simulink model "PriOrdemZero"  (R2015a)
settings: Solver=ode45  StartTime=0.0  StopTime=50  FixedStep=1e-8  RelTol=1e-5
settings Model: Creator=user  LastModifiedBy=user
settings SolverCC: ZeroCrossAlgorithm=Adaptive
settings OptimizationCC: BlockReduction=off  OptimizeBlockIOStorage=off  BufferReuse=off  GlobalBufferReuse=off  ExpressionFolding=off  LocalBlockOutputs=off
settings DebuggingCC: ConsistencyChecking=warning  UnderspecifiedInitializationDetection=Classic  MaxConsecutiveZCsMsg=warning  SolverPrmCheckMsg=warning

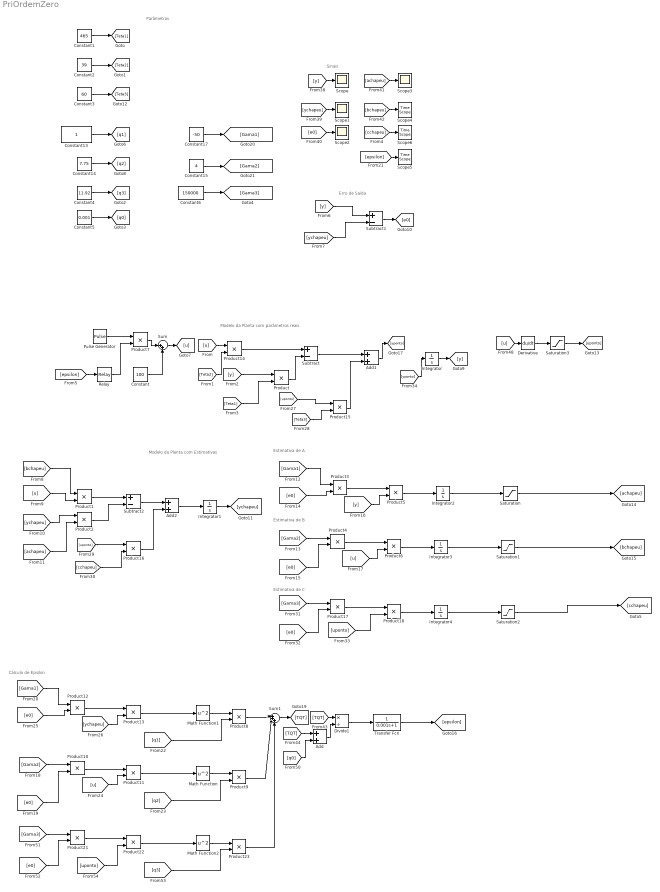
== system PriOrdemZero ==
  note: Cálculo de Epsilon
  note: Estimativa de B
  note: Estimativa de A
  note: Modelo da Planta com Estimativas
  note: Modelo da Planta com parâmetros reais
  note: Erro de Saída
  note: Parâmetros
  note: Sinais
  note: Estimativa de C
  Add : Sum  AccumDataTypeStr=double
  Add1 : Sum
  Add2 : Sum
  Constant : Constant  Value=100
  Constant1 : Constant  Value=465
  Constant13 : Constant
  Constant14 : Constant  Value=7.75
  Constant15 : Constant  Value=4
  Constant17 : Constant  Value=-50
  Constant2 : Constant  Value=39
  Constant3 : Constant  Value=60
  Constant4 : Constant  Value=11.92
  Constant5 : Constant  Value=0.001
  Constant6 : Constant  Value=150000
  Derivative : Derivative  CoefficientInTFapproximation=-1
  Divide1 : Product  Inputs=*/  OutDataTypeStr=double
  Integrator : Integrator
  Integrator1 : Integrator
  Integrator2 : Integrator  InitialCondition=70
  Integrator3 : Integrator  InitialCondition=80
  Integrator4 : Integrator  InitialCondition=78
  Math Function : Math  Operator=square  SaturateOnIntegerOverflow=on
  Math Function1 : Math  Operator=square  SaturateOnIntegerOverflow=on
  Math Function2 : Math  Operator=square  SaturateOnIntegerOverflow=on
  Product{,1..18,21..23} (22 alike) : Product
  Pulse Generator : DiscretePulseGenerator  PulseType=Time based  Amplitude=100  Period=0.01  PulseWidth=50
  Relay : Relay  OnSwitchValue=0.95  OffSwitchValue=0.05
  Saturation : Saturate  UpperLimit=500  LowerLimit=1
  Saturation1 : Saturate  UpperLimit=300  LowerLimit=1
  Saturation2 : Saturate  UpperLimit=3000  LowerLimit=0
  Saturation3 : Saturate  UpperLimit=10e6  LowerLimit=-10e6
  Scope{,1..3} (4 alike) : Scope
      Scope settings: YMin=9  YMax=16.5
      Scope1 settings: YMin=9  YMax=16.5  SampleInput=on
      Scope2 settings: YMin=-0.005  YMax=0.0045  SaveName=ScopeData2  SampleInput=on
      Scope3 settings: YMin=465.575  YMax=465.615  SaveName=ScopeData3  SampleInput=on
  Scope4 : TimeScope
  Scope5 : TimeScope
  Scope6 : TimeScope
  Subtract : Sum  Inputs=+-
  Subtract1 : Sum  Inputs=+-
  Subtract2 : Sum  Inputs=+-
  Sum : Sum  Inputs=|++
  Sum1 : Sum  Inputs=|+++
  Transfer Fcn : TransferFcn  Denominator=[0.001 1]
  wires:
  Constant/1 -> Sum/2
  [Teta2] -> Product14/2
  [Teta1] -> Product/2
  Product/1 -> Subtract/2
  Product14/1 -> Subtract/1
  Integrator/1 -> [y]
  [y] -> Product/1
  Sum/1 -> [u]
  [u] -> Product14/1
  [y] -> Subtract1/1
  [ychapeu] -> Subtract1/2
  Subtract1/1 -> [e0]
  Constant1/1 -> [Teta1]
  Constant2/1 -> [Teta2]
  Product1/1 -> Subtract2/1
  Product2/1 -> Subtract2/2
  [achapeu] -> Product2/2
  [ychapeu] -> Product2/1
  [u] -> Product1/2
  [bchapeu] -> Product1/1
  Integrator1/1 -> [ychapeu]
  [e0] -> Product3/2
  [Gama1] -> Product3/1
  [Gama2] -> Product4/1
  [e0] -> Product4/2
  Product4/1 -> Product6/1
  Product3/1 -> Product5/1
  [y] -> Product5/2
  [u] -> Product6/2
  Product5/1 -> Integrator2/1
  Product6/1 -> Integrator3/1
  Integrator3/1 -> Saturation1/1
  Integrator2/1 -> Saturation/1
  Product7/1 -> Sum/1
  Pulse Generator/1 -> Product7/1
  Product11/1 -> Math Function/1
  Product13/1 -> Math Function1/1
  Math Function1/1 -> Product8/1
  Math Function/1 -> Product9/1
  [q1] -> Product8/2
  [q2] -> Product9/2
  Product9/1 -> Sum1/2
  Product8/1 -> Sum1/1
  Constant13/1 -> [q1]
  Constant14/1 -> [q2]
  [y] -> Scope/1
  [ychapeu] -> Scope1/1
  [e0] -> Scope2/1
  [achapeu] -> Scope3/1
  [bchapeu] -> Scope4/1
  Constant17/1 -> [Gama1]
  Constant15/1 -> [Gama2]
  Add/1 -> Divide1/2
  [q0] -> Add/2
  Sum1/1 -> [TQT]
  [TQT] -> Divide1/1
  [TQT] -> Add/1
  [epsilon] -> Relay/1
  Saturation/1 -> [achapeu]
  Saturation1/1 -> [bchapeu]
  [Gama2] -> Product10/1
  [e0] -> Product10/2
  Product10/1 -> Product11/1
  [u] -> Product11/2
  [e0] -> Product12/2
  [Gama1] -> Product12/1
  Product12/1 -> Product13/1
  [ychapeu] -> Product13/2
  Relay/1 -> Product7/2
  [epsilon] -> Scope5/1
  Constant3/1 -> [Teta3]
  Constant4/1 -> [q3]
  Constant5/1 -> [q0]
  Constant6/1 -> [Gama3]
  [cchapeu] -> Scope6/1
  Subtract/1 -> Add1/1
  Product15/1 -> Add1/2
  [uponto] -> Product15/1
  [Teta3] -> Product15/2
  Subtract2/1 -> Add2/1
  Add2/1 -> Integrator1/1
  Product16/1 -> Add2/2
  [uponto] -> Product16/1
  [cchapeu] -> Product16/2
  [Gama3] -> Product17/1
  [e0] -> Product17/2
  Product17/1 -> Product18/1
  Product18/1 -> Integrator4/1
  Integrator4/1 -> Saturation2/1
  Saturation2/1 -> [cchapeu]
  [uponto] -> Product18/2
  Add1/1 -> [yponto]
  [yponto] -> Integrator/1
  [u] -> Derivative/1
  Derivative/1 -> Saturation3/1
  Saturation3/1 -> [uponto]
  Product22/1 -> Math Function2/1
  Math Function2/1 -> Product23/1
  [q3] -> Product23/2
  Product23/1 -> Sum1/3
  [Gama3] -> Product21/1
  [e0] -> Product21/2
  Product21/1 -> Product22/1
  [uponto] -> Product22/2
  Divide1/1 -> Transfer Fcn/1
  Transfer Fcn/1 -> [epsilon]
